simulink model "home_model"  (R2023b)
settings: Solver=VariableStepAuto  StartTime=0.0  StopTime=43200  MaxStep=0.05  RelTol=1e-3
libraries: SimscapeFluids_lib x32, fl_lib x31, nesl_utility x21
(part 1 of 2)
settings Model: Creator=jchouina  LastModifiedBy=jchouina

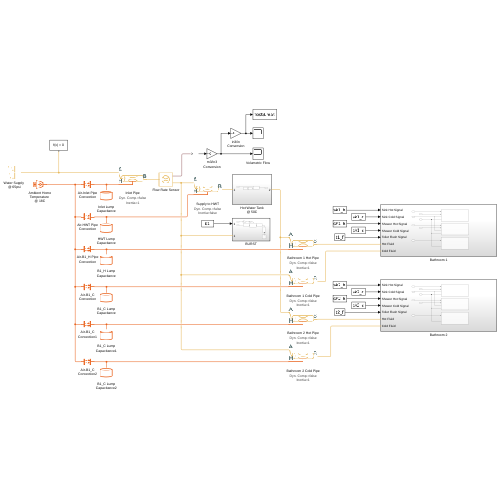
[thumbnail: Simulink's stored preview of the top-level diagram]
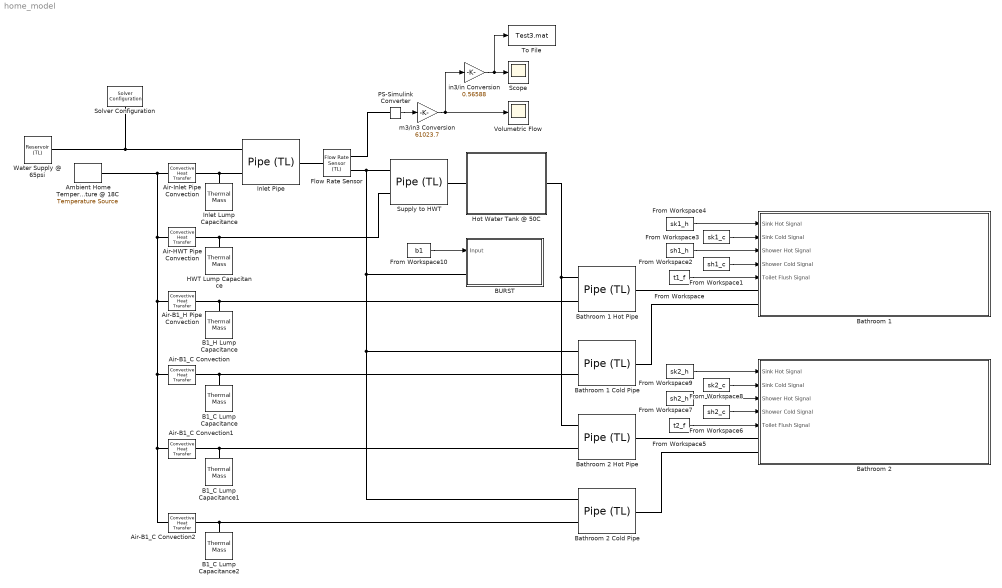
== system home_model ==
  Air-B1_C Convection : fl_lib/Thermal/Thermal Elements/Convective Heat Transfer  thermal_type=foundation.enum.constant_variable.constant  area=550 in^2  heat_tr_coeff=13.14 W/(K*m^2)  min_heat_tr_coeff=1e-3 W/(K*m^2)  T_specify=off  T_priority=None  T=0 K  T_nominal_specify=off  T_nominal_unit=K  T_nominal_value=1  Q_specify=off  Q_priority=None  Q=0 W  Q_nominal_specify=off  Q_nominal_unit=W  Q_nominal_value=1
  Air-B1_C Convection1 : fl_lib/Thermal/Thermal Elements/Convective Heat Transfer  thermal_type=foundation.enum.constant_variable.constant  area=550 in^2  heat_tr_coeff=13.14 W/(K*m^2)  min_heat_tr_coeff=1e-3 W/(K*m^2)  T_specify=off  T_priority=None  T=0 K  T_nominal_specify=off  T_nominal_unit=K  T_nominal_value=1  Q_specify=off  Q_priority=None  Q=0 W  Q_nominal_specify=off  Q_nominal_unit=W  Q_nominal_value=1
  Air-B1_C Convection2 : fl_lib/Thermal/Thermal Elements/Convective Heat Transfer  thermal_type=foundation.enum.constant_variable.constant  area=550 in^2  heat_tr_coeff=13.14 W/(K*m^2)  min_heat_tr_coeff=1e-3 W/(K*m^2)  T_specify=off  T_priority=None  T=0 K  T_nominal_specify=off  T_nominal_unit=K  T_nominal_value=1  Q_specify=off  Q_priority=None  Q=0 W  Q_nominal_specify=off  Q_nominal_unit=W  Q_nominal_value=1
  Air-B1_H Pipe Convection : fl_lib/Thermal/Thermal Elements/Convective Heat Transfer  thermal_type=foundation.enum.constant_variable.constant  area=550 in^2  heat_tr_coeff=13.14 W/(K*m^2)  min_heat_tr_coeff=1e-3 W/(K*m^2)  T_specify=off  T_priority=None  T=0 K  T_nominal_specify=off  T_nominal_unit=K  T_nominal_value=1  Q_specify=off  Q_priority=None  Q=0 W  Q_nominal_specify=off  Q_nominal_unit=W  Q_nominal_value=1
  Air-HWT Pipe Convection : fl_lib/Thermal/Thermal Elements/Convective Heat Transfer  thermal_type=foundation.enum.constant_variable.constant  area=550 in^2  heat_tr_coeff=13.14 W/(K*m^2)  min_heat_tr_coeff=1e-3 W/(K*m^2)  T_specify=off  T_priority=None  T=0 K  T_nominal_specify=off  T_nominal_unit=K  T_nominal_value=1  Q_specify=off  Q_priority=None  Q=0 W  Q_nominal_specify=off  Q_nominal_unit=W  Q_nominal_value=1
  Air-Inlet Pipe Convection : fl_lib/Thermal/Thermal Elements/Convective Heat Transfer  thermal_type=foundation.enum.constant_variable.constant  area=550 in^2  heat_tr_coeff=13.14 W/(K*m^2)  min_heat_tr_coeff=1e-3 W/(K*m^2)  T_specify=off  T_priority=None  T=0 K  T_nominal_specify=off  T_nominal_unit=K  T_nominal_value=1  Q_specify=off  Q_priority=None  Q=0 W  Q_nominal_specify=off  Q_nominal_unit=W  Q_nominal_value=1
  Ambient Home Temperature @ 18C : fl_lib/Thermal/Thermal Sources/Temperature Source  temperature=18 degC
  B1_C Lump Capacitance : fl_lib/Thermal/Thermal Elements/Thermal Mass  mass_type=foundation.enum.constant_variable.constant  mass=2.25 kg  sp_heat=390 J/(K*kg)  mass_min=1e-6 kg  num_ports=foundation.enum.numPorts2.one  m_specify=off  m_priority=High  m=1 kg  m_nominal_specify=off  m_nominal_unit=kg  m_nominal_value=1  T_specify=off  T_priority=High  T=300 K  T_nominal_specify=off  T_nominal_unit=K  T_nominal_value=1  Q_specify=off  Q_priority=None  Q=0 W  Q_nominal_specify=off  Q_nominal_unit=W  Q_nominal_value=1
  B1_C Lump Capacitance1 : fl_lib/Thermal/Thermal Elements/Thermal Mass  mass_type=foundation.enum.constant_variable.constant  mass=2.25 kg  sp_heat=390 J/(K*kg)  mass_min=1e-6 kg  num_ports=foundation.enum.numPorts2.one  m_specify=off  m_priority=High  m=1 kg  m_nominal_specify=off  m_nominal_unit=kg  m_nominal_value=1  T_specify=off  T_priority=High  T=300 K  T_nominal_specify=off  T_nominal_unit=K  T_nominal_value=1  Q_specify=off  Q_priority=None  Q=0 W  Q_nominal_specify=off  Q_nominal_unit=W  Q_nominal_value=1
  B1_C Lump Capacitance2 : fl_lib/Thermal/Thermal Elements/Thermal Mass  mass_type=foundation.enum.constant_variable.constant  mass=2.25 kg  sp_heat=390 J/(K*kg)  mass_min=1e-6 kg  num_ports=foundation.enum.numPorts2.one  m_specify=off  m_priority=High  m=1 kg  m_nominal_specify=off  m_nominal_unit=kg  m_nominal_value=1  T_specify=off  T_priority=High  T=300 K  T_nominal_specify=off  T_nominal_unit=K  T_nominal_value=1  Q_specify=off  Q_priority=None  Q=0 W  Q_nominal_specify=off  Q_nominal_unit=W  Q_nominal_value=1
  B1_H Lump Capacitance : fl_lib/Thermal/Thermal Elements/Thermal Mass  mass_type=foundation.enum.constant_variable.constant  mass=2.25 kg  sp_heat=390 J/(K*kg)  mass_min=1e-6 kg  num_ports=foundation.enum.numPorts2.one  m_specify=off  m_priority=High  m=1 kg  m_nominal_specify=off  m_nominal_unit=kg  m_nominal_value=1  T_specify=off  T_priority=High  T=300 K  T_nominal_specify=off  T_nominal_unit=K  T_nominal_value=1  Q_specify=off  Q_priority=None  Q=0 W  Q_nominal_specify=off  Q_nominal_unit=W  Q_nominal_value=1
  BURST : Subsystem
  Bathroom 1 : Subsystem
  Bathroom 1 Cold Pipe : fl_lib/Thermal Liquid/Elements/Pipe (TL)  length=360 in  area=0.442 in^2  Dh=0.75 in  length_add=0 m  roughness=1e-5 m  Re_lam=2000  Re_tur=4000  shape_factor=64  Nu_lam=3.66  dynamic_compressibility=false  inertia=1  p0=65 psi  T0=283.15 K  mdot0=0 kg/s
      settings: AttributesFormatString=|
      | Dyn. Comp.=%<dynamic_compressibility>
      | Inertia=%<inertia>
  Bathroom 1 Hot Pipe : fl_lib/Thermal Liquid/Elements/Pipe (TL)  length=360 in  area=0.442 in^2  Dh=0.75 in  length_add=0 m  roughness=1e-5 m  Re_lam=2000  Re_tur=4000  shape_factor=64  Nu_lam=3.66  dynamic_compressibility=false  inertia=1  p0=65 psi  T0=283.15 K  mdot0=0 kg/s
      settings: AttributesFormatString=|
      | Dyn. Comp.=%<dynamic_compressibility>
      | Inertia=%<inertia>
  Bathroom 2 : Subsystem
  Bathroom 2 Cold Pipe : fl_lib/Thermal Liquid/Elements/Pipe (TL)  length=440 in  area=0.442 in^2  Dh=0.75 in  length_add=0 m  roughness=1e-5 m  Re_lam=2000  Re_tur=4000  shape_factor=64  Nu_lam=3.66  dynamic_compressibility=false  inertia=1  p0=65 psi  T0=283.15 K  mdot0=0 kg/s
      settings: AttributesFormatString=|
      | Dyn. Comp.=%<dynamic_compressibility>
      | Inertia=%<inertia>
  Bathroom 2 Hot Pipe : fl_lib/Thermal Liquid/Elements/Pipe (TL)  length=440 in  area=0.442 in^2  Dh=0.75 in  length_add=0 m  roughness=1e-5 m  Re_lam=2000  Re_tur=4000  shape_factor=64  Nu_lam=3.66  dynamic_compressibility=false  inertia=1  p0=65 psi  T0=283.15 K  mdot0=0 kg/s
      settings: AttributesFormatString=|
      | Dyn. Comp.=%<dynamic_compressibility>
      | Inertia=%<inertia>
  "Flow Rate Sensor " : fl_lib/Thermal Liquid/Sensors/Flow Rate Sensor (TL)  mass_flow_measure=false  volumetric_flow_measure=true  energy_flow_measure=false
      settings: InternalSimscapePortConfiguration="{\"Bottom\":[],\"Left\":[{\"id\":\"A\",\"label\":\"A\",\"type\":\"foundation.thermal_liquid.thermal_liquid\"}],\"Right\":[{\"id\":\"B\",\"label\":\"B\",\"type\":\"foundation.thermal_liquid.thermal_liquid\"},{\"id\":\"V\",\"label\":\"V\",\"type\":\"output\"}],\"Top\":[]}"
  From Workspace : FromWorkspace  VariableName=t1_f  SampleTime=-1
  From Workspace1 : FromWorkspace  VariableName=sh1_c  SampleTime=-1
  From Workspace10 : FromWorkspace  VariableName=b1
  From Workspace2 : FromWorkspace  VariableName=sh1_h  SampleTime=-1
  From Workspace3 : FromWorkspace  VariableName=sk1_c  SampleTime=-1
  From Workspace4 : FromWorkspace  VariableName=sk1_h  SampleTime=-1
  From Workspace5 : FromWorkspace  VariableName=t2_f  SampleTime=-1
  From Workspace6 : FromWorkspace  VariableName=sh2_c  SampleTime=-1
  From Workspace7 : FromWorkspace  VariableName=sh2_h  SampleTime=-1
  From Workspace8 : FromWorkspace  VariableName=sk2_c  SampleTime=-1
  From Workspace9 : FromWorkspace  VariableName=sk2_h  SampleTime=-1
  HWT Lump Capacitance : fl_lib/Thermal/Thermal Elements/Thermal Mass  mass_type=foundation.enum.constant_variable.constant  mass=2.25 kg  sp_heat=390 J/(K*kg)  mass_min=1e-6 kg  num_ports=foundation.enum.numPorts2.one  m_specify=off  m_priority=High  m=1 kg  m_nominal_specify=off  m_nominal_unit=kg  m_nominal_value=1  T_specify=off  T_priority=High  T=300 K  T_nominal_specify=off  T_nominal_unit=K  T_nominal_value=1  Q_specify=off  Q_priority=None  Q=0 W  Q_nominal_specify=off  Q_nominal_unit=W  Q_nominal_value=1
  Hot Water Tank @ 50C : Subsystem
  Inlet Lump Capacitance : fl_lib/Thermal/Thermal Elements/Thermal Mass  mass_type=foundation.enum.constant_variable.constant  mass=4.5 kg  sp_heat=390 J/(K*kg)  mass_min=1e-6 kg  num_ports=foundation.enum.numPorts2.one  m_specify=off  m_priority=High  m=1 kg  m_nominal_specify=off  m_nominal_unit=kg  m_nominal_value=1  T_specify=off  T_priority=High  T=300 K  T_nominal_specify=off  T_nominal_unit=K  T_nominal_value=1  Q_specify=off  Q_priority=None  Q=0 W  Q_nominal_specify=off  Q_nominal_unit=W  Q_nominal_value=1
  Inlet Pipe : fl_lib/Thermal Liquid/Elements/Pipe (TL)  length=200 in  area=0.442 in^2  Dh=0.75 in  length_add=0 m  roughness=1e-5 m  Re_lam=2000  Re_tur=4000  shape_factor=64  Nu_lam=3.66  dynamic_compressibility=false  inertia=1  p0=65 psi  T0=283.15 K  mdot0=0 kg/s
      settings: AttributesFormatString=|
      | Dyn. Comp.=%<dynamic_compressibility>
      | Inertia=%<inertia>
  PS-Simulink Converter : nesl_utility/PS-Simulink Converter  PhysicalDomain=network_engine_domain  SubClassName=ps_output  LeftPortType=input  RightPortType=output  PseudoPeriodic=off  Frequencies=[]  VectorFormat=inherit  Unit=inherit  AffineConversion=off
  Scope : Scope
  Solver Configuration : nesl_utility/Solver Configuration  PhysicalDomain=network_engine_domain  SubClassName=solver  LeftPortType=input  RightPortType=generic  Tones=[]  Harmonics=[]  SimulateNoise=off  Profile=off  UseLocalSampling=off  EnableSwitchedLinearOptims=on  FrequencyDomain=off  UseCCode=off  RelTol=0.001  AbsTol=0.001  MinStep=1e-09  ToWorkspace=off  RevertToSquareIcSolve=off  NumHomotopyIterations=100  PhasorMode=off  PhasorModeNumHarmonics=1  ConsistencySolver=NEWTON_XTOL_AFTER_FTOL  IndexReductionMethod=DerivativeReplacement  DoDC=off  ResidualTolerance=1e-09  ConsistencyTolSource=GLOBAL  ConsistencyAbsTol=0.001  ConsistencyRelTol=0.001  ConsistencyTolFactor=0.001  UseLocalSolver=off  LocalSolverChoice=NE_BACKWARD_EULER_ADVANCER  ResolveIndetEquations=on  FunctionEvalNumThread=1  LocalSolverSampleTime=0.001  DoFixedCost=off  MaxNonlinIter=3  MaxModeIter=2  ComputeImpulses=off  ImpulseIterations=2  LinearAlgebra=auto  LinearAlgebraNumThread=0  EquationFormulation=NE_TIME_EF  DelaysMemoryBudget=1024  AutomaticFiltering=on  FilteringTimeConstant=0.001  PartitionStorageMethod=AS_NEEDED  PartitionMemoryBudget=1024  PartitionMethod=ROBUST  MultibodyUseLocalSolver=off  MultibodyLocalSolverChoice=ODE1  MultibodyLocalSolverSampleTime=0.001
  Supply to HWT : fl_lib/Thermal Liquid/Elements/Pipe (TL)  length=100 in  area=0.442 in^2  Dh=0.75 in  length_add=0 m  roughness=1e-5 m  Re_lam=2000  Re_tur=4000  shape_factor=64  Nu_lam=3.66  dynamic_compressibility=false  inertia=false  p0=1 atm  T0=283.15 K  mdot0=0 kg/s
      settings: AttributesFormatString=|
      | Dyn. Comp.=%<dynamic_compressibility>
      | Inertia=%<inertia>
  To File : ToFile  Filename=Test3.mat  MatrixName=linRate  SaveFormat=Timeseries
  Volumetric Flow : Scope
  Water Supply @ 65psi : fl_lib/Thermal Liquid/Elements/Reservoir (TL)  pressure_spec=foundation.enum.pressure_spec.specified  reservoir_pressure=65 psi  reservoir_temperature=283.15 K  area=0.442 in^2
  in3/in Conversion : Gain  Gain=0.56588
  m3/in3 Conversion : Gain  Gain=61023.7
  wires:
  From Workspace/1 -> Bathroom 1/5(Toilet Flush Signal)
  From Workspace1/1 -> Bathroom 1/4(Shower Cold Signal)
  From Workspace2/1 -> Bathroom 1/3(Shower Hot Signal)
  From Workspace4/1 -> Bathroom 1/1(Sink Hot Signal)
  From Workspace3/1 -> Bathroom 1/2(Sink Cold Signal)
  From Workspace9/1 -> Bathroom 2/1(Sink Hot Signal)
  From Workspace7/1 -> Bathroom 2/3(Shower Hot Signal)
  From Workspace6/1 -> Bathroom 2/4(Shower Cold Signal)
  From Workspace8/1 -> Bathroom 2/2(Sink Cold Signal)
  From Workspace5/1 -> Bathroom 2/5(Toilet Flush Signal)
  PS-Simulink Converter/1 -> m3/in3 Conversion/1
  m3/in3 Conversion/1 -> in3/in Conversion/1, Volumetric Flow/1
  in3/in Conversion/1 -> To File/1, Scope/1
  From Workspace10/1 -> BURST/1(Input)
  connections:
  Air-Inlet Pipe Convection/RConn1 -- Inlet Pipe/LConn2 -- Inlet Lump Capacitance/LConn1
  Water Supply @ 65psi/LConn1 -- Solver Configuration/RConn1 -- Inlet Pipe/LConn1
  "Flow Rate Sensor "/LConn1 -- Inlet Pipe/RConn1
  PS-Simulink Converter/LConn1 -- "Flow Rate Sensor "/RConn2
  Air-Inlet Pipe Convection/LConn1 -- Air-B1_H Pipe Convection/LConn1 -- Air-B1_C Convection/LConn1 -- Air-B1_C Convection1/LConn1 -- Air-B1_C Convection2/LConn1 -- Air-HWT Pipe Convection/LConn1 -- Ambient Home Temperature @ 18C/LConn1
  Bathroom 1 Cold Pipe/LConn1 -- Supply to HWT/LConn1 -- "Flow Rate Sensor "/RConn1 -- BURST/LConn1 -- Bathroom 2 Cold Pipe/LConn1
  Supply to HWT/LConn2 -- Air-HWT Pipe Convection/RConn1 -- HWT Lump Capacitance/LConn1
  Bathroom 1/LConn2 -- Bathroom 1 Cold Pipe/RConn1
  Air-B1_C Convection/RConn1 -- B1_C Lump Capacitance/LConn1 -- Bathroom 1 Cold Pipe/LConn2
  Bathroom 1 Hot Pipe/LConn1 -- Hot Water Tank @ 50C/RConn1 -- Bathroom 2 Hot Pipe/LConn1
  Air-B1_H Pipe Convection/RConn1 -- Bathroom 1 Hot Pipe/LConn2 -- B1_H Lump Capacitance/LConn1
  Bathroom 1 Hot Pipe/RConn1 -- Bathroom 1/LConn1
  Hot Water Tank @ 50C/LConn1 -- Supply to HWT/RConn1
  B1_C Lump Capacitance1/LConn1 -- Bathroom 2 Hot Pipe/LConn2 -- Air-B1_C Convection1/RConn1
  B1_C Lump Capacitance2/LConn1 -- Bathroom 2 Cold Pipe/LConn2 -- Air-B1_C Convection2/RConn1
  Bathroom 2/LConn2 -- Bathroom 2 Cold Pipe/RConn1
  Bathroom 2/LConn1 -- Bathroom 2 Hot Pipe/RConn1

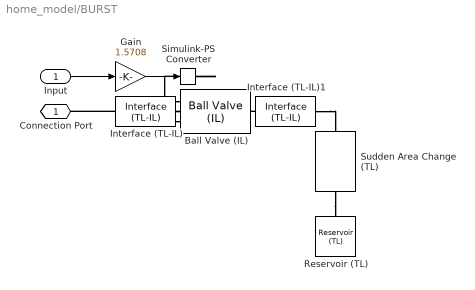
== system home_model/BURST ==
  Input : Inport
  Ball Valve (IL) : SimscapeFluids_lib/Isothermal Liquid/Valves & Orifices/Flow Control Valves/Ball Valve (IL)  valve_type=fluids.isothermal_liquid.valves_orifices.flow_control_valves.enum.BallValveSpec.Standard  parameterization=fluids.isothermal_liquid.valves_orifices.flow_control_valves.enum.FlowCoefficientSpec.Kv  Cv_max=32 gpm  Kv_max=49 m^3/hr  Cd=0.64  area_port=pi * (25 ^ 2) / 4 mm^2  area_ball=pi * (20 ^ 2) / 4 mm^2  Cv_TLU=[1e-06, .58, 1.15, 1.9, 2.8, 4.3, 7, 10.5, 17, 26, 32] gpm  Kv_TLU=[1e-06, .34, .76, 1.6, 2.45, 4.1, 5.75, 9.4, 13, 28, 50] m^3/hr  area_TLU=[1e-10, 62.5, 125, 187.5, 250, 312.5, 375, 437.5, 500, 562.5, 625] mm^2  rotation_TLU=pi / 2 .* [0, .1, .2, .3, .4, .5, .6, .7, .8, .9, 1] rad  area_leak=1e-10 m^2  Re_c=150  rho_water60F=0.99897 g/cm^3  rho_water15C=0.99913 g/cm^3
      settings: InternalSimscapePortConfiguration="{\"Bottom\":[],\"Left\":[{\"id\":\"A\",\"label\":\"A\",\"type\":\"foundation.isothermal_liquid.isothermal_liquid\"}],\"Right\":[{\"id\":\"B\",\"label\":\"B\",\"type\":\"foundation.isothermal_liquid.isothermal_liquid\"}],\"Top\":[{\"id\":\"S\",\"label\":\"S\",\"type\":\"input\"}]}"
  Gain : Gain  Gain=1.5708
  Interface (TL-IL) : SimscapeFluids_lib/Fluid Network Interfaces/Interface (TL-IL)  interface_domain_spec=fluids.interfaces.enum.interface_domain_spec.TL_IL  temperature_spec=foundation.enum.constant_controlled.constant  T_interface=293.15 K  area_TL=0.01 m^2
      settings: InternalSimscapePortConfiguration="{\"Bottom\":[],\"Left\":[{\"id\":\"TL\",\"label\":\"TL\",\"type\":\"foundation.thermal_liquid.thermal_liquid\"}],\"Right\":[{\"id\":\"IL\",\"label\":\"IL\",\"type\":\"foundation.isothermal_liquid.isothermal_liquid\"}],\"Top\":[]}"
  Interface (TL-IL)1 : SimscapeFluids_lib/Fluid Network Interfaces/Interface (TL-IL)  interface_domain_spec=fluids.interfaces.enum.interface_domain_spec.TL_IL  temperature_spec=foundation.enum.constant_controlled.constant  T_interface=293.15 K  area_TL=0.01 m^2
      settings: InternalSimscapePortConfiguration="{\"Bottom\":[],\"Left\":[{\"id\":\"TL\",\"label\":\"TL\",\"type\":\"foundation.thermal_liquid.thermal_liquid\"}],\"Right\":[{\"id\":\"IL\",\"label\":\"IL\",\"type\":\"foundation.isothermal_liquid.isothermal_liquid\"}],\"Top\":[]}"
  Reservoir (TL) : fl_lib/Thermal Liquid/Elements/Reservoir (TL)  pressure_spec=foundation.enum.pressure_spec.atmospheric  reservoir_pressure=0.101325 MPa  reservoir_temperature=293.15 K  area=0.01 m^2
  Simulink-PS Converter : nesl_utility/Simulink-PS Converter  PhysicalDomain=network_engine_domain  SubClassName=ps_input  LeftPortType=input  RightPortType=output  PseudoPeriodic=off  Frequencies=[]  NoiseDistribution=none  NoiseParameters=[]  Unit=1  AffineConversion=off  FilteringAndDerivatives=provide  SimscapeFilterOrder=1  InputFilterTimeConstant=0.001  UdotUserProvided=0
  Sudden Area Change (TL) : SimscapeFluids_lib/Thermal Liquid/Pipes & Fittings/Sudden Area Change (TL)  loss_spec=fluids.thermal_liquid.enum.area_change_loss_spec.empirical  area_A=0.442 m^2  area_B=10 in^2  K_c=1  K_e=1  Re_TLU=[10, 20, 30, 40, 50, 100, 200, 500, 1000, 2000]  loss_contraction_TLU=[5, 2.7, 1.8, 1.46, 1.3, .9, .65, .42, .3, .2]  loss_expansion_TLU=[3.1, 2.3, 1.65, 1.35, 1.15, .9, .75, .65, .9, .65]  Re_critical=150
      settings: InternalSimscapePortConfiguration="{\"Bottom\":[],\"Left\":[{\"id\":\"A\",\"label\":\"A\",\"type\":\"foundation.thermal_liquid.thermal_liquid\"}],\"Right\":[{\"id\":\"B\",\"label\":\"B\",\"type\":\"foundation.thermal_liquid.thermal_liquid\"}],\"Top\":[]}"
  Connection Port : PMIOPort  Side=Left
  wires:
  Input/1 -> Gain/1
  Gain/1 -> Simulink-PS Converter/1
  connections:
  Interface (TL-IL)/RConn1 -- Ball Valve (IL)/LConn1
  Simulink-PS Converter/RConn1 -- Ball Valve (IL)/LConn2
  Interface (TL-IL)/LConn1 -- Connection Port/RConn1
  Sudden Area Change (TL)/RConn1 -- Reservoir (TL)/LConn1
  Interface (TL-IL)1/LConn1 -- Sudden Area Change (TL)/LConn1
  Interface (TL-IL)1/RConn1 -- Ball Valve (IL)/RConn1

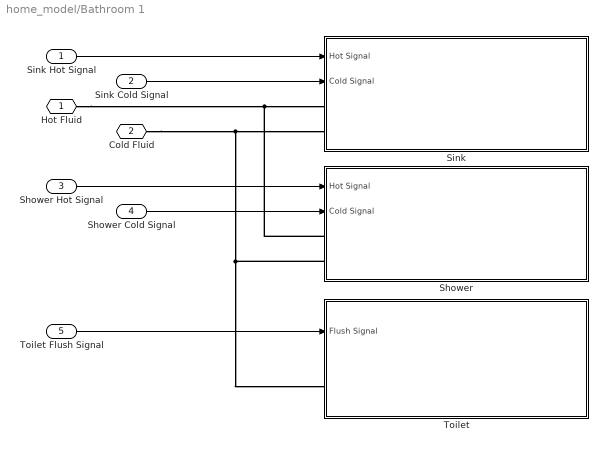
== system home_model/Bathroom 1 ==
  Sink Hot Signal : Inport
  Sink Cold Signal : Inport  Port=2
  Shower Hot Signal : Inport  Port=3
  Shower Cold Signal : Inport  Port=4
  Toilet Flush Signal : Inport  Port=5
  Shower : Subsystem
  Sink : Subsystem
  Toilet : Subsystem
  Hot Fluid : PMIOPort  Side=Left
  Cold Fluid : PMIOPort  Port=2  Side=Left
  wires:
  Sink Hot Signal/1 -> Sink/1(Hot Signal)
  Sink Cold Signal/1 -> Sink/2(Cold Signal)
  Shower Cold Signal/1 -> Shower/2(Cold Signal)
  Shower Hot Signal/1 -> Shower/1(Hot Signal)
  Toilet Flush Signal/1 -> Toilet/1(Flush Signal)
  connections:
  Hot Fluid/RConn1 -- Shower/LConn1 -- Sink/LConn1
  Cold Fluid/RConn1 -- Sink/LConn2 -- Toilet/LConn1 -- Shower/LConn2

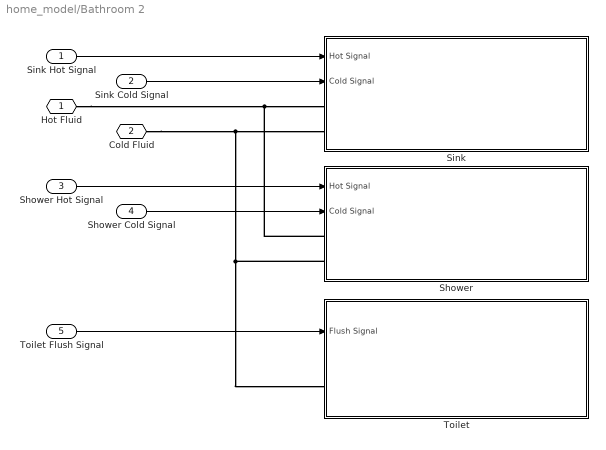
== system home_model/Bathroom 2 ==
  Sink Hot Signal : Inport
  Sink Cold Signal : Inport  Port=2
  Shower Hot Signal : Inport  Port=3
  Shower Cold Signal : Inport  Port=4
  Toilet Flush Signal : Inport  Port=5
  Shower : Subsystem
  Sink : Subsystem
  Toilet : Subsystem
  Hot Fluid : PMIOPort  Side=Left
  Cold Fluid : PMIOPort  Port=2  Side=Left
  wires:
  Sink Hot Signal/1 -> Sink/1(Hot Signal)
  Sink Cold Signal/1 -> Sink/2(Cold Signal)
  Shower Cold Signal/1 -> Shower/2(Cold Signal)
  Shower Hot Signal/1 -> Shower/1(Hot Signal)
  Toilet Flush Signal/1 -> Toilet/1(Flush Signal)
  connections:
  Hot Fluid/RConn1 -- Shower/LConn1 -- Sink/LConn1
  Cold Fluid/RConn1 -- Sink/LConn2 -- Toilet/LConn1 -- Shower/LConn2

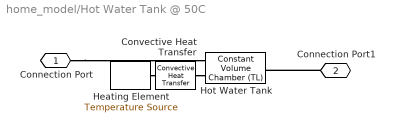
== system home_model/Hot Water Tank @ 50C ==
  Convective Heat Transfer : fl_lib/Thermal/Thermal Elements/Convective Heat Transfer  thermal_type=foundation.enum.constant_variable.constant  area=0.135 m^2  heat_tr_coeff=800 W/(K*m^2)  min_heat_tr_coeff=1e-3 W/(K*m^2)  T_specify=off  T_priority=None  T=0 K  T_nominal_specify=off  T_nominal_unit=K  T_nominal_value=1  Q_specify=off  Q_priority=None  Q=0 W  Q_nominal_specify=off  Q_nominal_unit=W  Q_nominal_value=1
  Heating Element : fl_lib/Thermal/Thermal Sources/Temperature Source  temperature=50 degC
  Hot Water Tank : fl_lib/Thermal Liquid/Elements/Constant Volume Chamber (TL)  volume=40 gal  num_ports=foundation.enum.num_ports.two  area_A=0.442 in^2  area_B=0.442 in^2  area_C=0.01 m^2  area_D=0.01 m^2  p_I_specify=off  p_I_priority=High  p_I=0.101325 MPa  p_I_nominal_specify=off  p_I_nominal_unit=MPa  p_I_nominal_value=1  T_I_specify=off  T_I_priority=High  T_I=293.15 K  T_I_nominal_specify=off  T_I_nominal_unit=K  T_I_nominal_value=1  u_I_specify=off  u_I_priority=None  u_I=83.906 kJ/kg  u_I_nominal_specify=off  u_I_nominal_unit=kJ/kg  u_I_nominal_value=1  rho_I_specify=off  rho_I_priority=None  rho_I=998.21 kg/m^3  rho_I_nominal_specify=off  rho_I_nominal_unit=kg/m^3  rho_I_nominal_value=1
      settings: InternalSimscapePortConfiguration="{\"Bottom\":[],\"Left\":[{\"id\":\"A\",\"label\":\"A\",\"type\":\"foundation.thermal_liquid.thermal_liquid\"},{\"id\":\"H\",\"label\":\"H\",\"type\":\"foundation.thermal.thermal\"}],\"Right\":[{\"id\":\"B\",\"label\":\"B\",\"type\":\"foundation.thermal_liquid.thermal_liquid\"}],\"Top\":[]}"
  Connection Port : PMIOPort  Side=Left
  Connection Port1 : PMIOPort  Port=2  Side=Right
  connections:
  Heating Element/LConn1 -- Convective Heat Transfer/LConn1
  Convective Heat Transfer/RConn1 -- Hot Water Tank/LConn2
  Connection Port/RConn1 -- Hot Water Tank/LConn1
  Connection Port1/RConn1 -- Hot Water Tank/RConn1

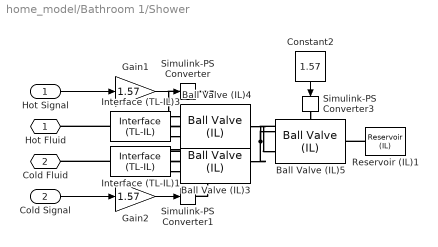
== system home_model/Bathroom 1/Shower ==
  Hot Signal : Inport
  Cold Signal : Inport  Port=2
  Ball Valve (IL)3 : SimscapeFluids_lib/Isothermal Liquid/Valves & Orifices/Flow Control Valves/Ball Valve (IL)  valve_type=fluids.isothermal_liquid.valves_orifices.flow_control_valves.enum.BallValveSpec.Standard  parameterization=fluids.isothermal_liquid.valves_orifices.flow_control_valves.enum.FlowCoefficientSpec.Kv  Cv_max=32 gpm  Kv_max=2 gpm  Cd=0.64  area_port=pi * (75 ^ 2) / 4 mm^2  area_ball=pi * (75 ^ 2) / 4 mm^2  Cv_TLU=[1e-06, .58, 1.15, 1.9, 2.8, 4.3, 7, 10.5, 17, 26, 32] gpm  Kv_TLU=[1e-06, .34, .76, 1.6, 2.45, 4.1, 5.75, 9.4, 13, 28, 50] m^3/hr  area_TLU=[1e-10, 62.5, 125, 187.5, 250, 312.5, 375, 437.5, 500, 562.5, 625] mm^2  rotation_TLU=pi / 2 .* [0, .1, .2, .3, .4, .5, .6, .7, .8, .9, 1] rad  area_leak=1e-10 m^2  Re_c=150  rho_water60F=0.99897 g/cm^3  rho_water15C=0.99913 g/cm^3
      settings: InternalSimscapePortConfiguration="{\"Bottom\":[],\"Left\":[{\"id\":\"A\",\"label\":\"A\",\"type\":\"foundation.isothermal_liquid.isothermal_liquid\"}],\"Right\":[{\"id\":\"B\",\"label\":\"B\",\"type\":\"foundation.isothermal_liquid.isothermal_liquid\"}],\"Top\":[{\"id\":\"S\",\"label\":\"S\",\"type\":\"input\"}]}"
  Ball Valve (IL)4 : SimscapeFluids_lib/Isothermal Liquid/Valves & Orifices/Flow Control Valves/Ball Valve (IL)  valve_type=fluids.isothermal_liquid.valves_orifices.flow_control_valves.enum.BallValveSpec.Standard  parameterization=fluids.isothermal_liquid.valves_orifices.flow_control_valves.enum.FlowCoefficientSpec.Kv  Cv_max=32 gpm  Kv_max=2 gpm  Cd=0.64  area_port=pi * (75 ^ 2) / 4 mm^2  area_ball=pi * (75 ^ 2) / 4 mm^2  Cv_TLU=[1e-06, .58, 1.15, 1.9, 2.8, 4.3, 7, 10.5, 17, 26, 32] gpm  Kv_TLU=[1e-06, .34, .76, 1.6, 2.45, 4.1, 5.75, 9.4, 13, 28, 50] m^3/hr  area_TLU=[1e-10, 62.5, 125, 187.5, 250, 312.5, 375, 437.5, 500, 562.5, 625] mm^2  rotation_TLU=pi / 2 .* [0, .1, .2, .3, .4, .5, .6, .7, .8, .9, 1] rad  area_leak=1e-10 m^2  Re_c=150  rho_water60F=0.99897 g/cm^3  rho_water15C=0.99913 g/cm^3
      settings: InternalSimscapePortConfiguration="{\"Bottom\":[],\"Left\":[{\"id\":\"A\",\"label\":\"A\",\"type\":\"foundation.isothermal_liquid.isothermal_liquid\"}],\"Right\":[{\"id\":\"B\",\"label\":\"B\",\"type\":\"foundation.isothermal_liquid.isothermal_liquid\"}],\"Top\":[{\"id\":\"S\",\"label\":\"S\",\"type\":\"input\"}]}"
  Ball Valve (IL)5 : SimscapeFluids_lib/Isothermal Liquid/Valves & Orifices/Flow Control Valves/Ball Valve (IL)  valve_type=fluids.isothermal_liquid.valves_orifices.flow_control_valves.enum.BallValveSpec.Standard  parameterization=fluids.isothermal_liquid.valves_orifices.flow_control_valves.enum.FlowCoefficientSpec.Kv  Cv_max=32 gpm  Kv_max=2 gpm  Cd=0.64  area_port=pi * (25 ^ 2) / 4 mm^2  area_ball=pi * (20 ^ 2) / 4 mm^2  Cv_TLU=[1e-06, .58, 1.15, 1.9, 2.8, 4.3, 7, 10.5, 17, 26, 32] gpm  Kv_TLU=[1e-06, .34, .76, 1.6, 2.45, 4.1, 5.75, 9.4, 13, 28, 50] m^3/hr  area_TLU=[1e-10, 62.5, 125, 187.5, 250, 312.5, 375, 437.5, 500, 562.5, 625] mm^2  rotation_TLU=pi / 2 .* [0, .1, .2, .3, .4, .5, .6, .7, .8, .9, 1] rad  area_leak=1e-10 m^2  Re_c=150  rho_water60F=0.99897 g/cm^3  rho_water15C=0.99913 g/cm^3
      settings: InternalSimscapePortConfiguration="{\"Bottom\":[],\"Left\":[{\"id\":\"A\",\"label\":\"A\",\"type\":\"foundation.isothermal_liquid.isothermal_liquid\"}],\"Right\":[{\"id\":\"B\",\"label\":\"B\",\"type\":\"foundation.isothermal_liquid.isothermal_liquid\"}],\"Top\":[{\"id\":\"S\",\"label\":\"S\",\"type\":\"input\"}]}"
  Constant2 : Constant  Value=1.57
  Gain1 : Gain  Gain=1.57
  Gain2 : Gain  Gain=1.57
  Interface (TL-IL)1 : SimscapeFluids_lib/Fluid Network Interfaces/Interface (TL-IL)  interface_domain_spec=fluids.interfaces.enum.interface_domain_spec.TL_IL  temperature_spec=foundation.enum.constant_controlled.constant  T_interface=293.15 K  area_TL=0.01 m^2
      settings: InternalSimscapePortConfiguration="{\"Bottom\":[],\"Left\":[{\"id\":\"TL\",\"label\":\"TL\",\"type\":\"foundation.thermal_liquid.thermal_liquid\"}],\"Right\":[{\"id\":\"IL\",\"label\":\"IL\",\"type\":\"foundation.isothermal_liquid.isothermal_liquid\"}],\"Top\":[]}"
  Interface (TL-IL)3 : SimscapeFluids_lib/Fluid Network Interfaces/Interface (TL-IL)  interface_domain_spec=fluids.interfaces.enum.interface_domain_spec.TL_IL  temperature_spec=foundation.enum.constant_controlled.constant  T_interface=293.15 K  area_TL=0.01 m^2
      settings: InternalSimscapePortConfiguration="{\"Bottom\":[],\"Left\":[{\"id\":\"TL\",\"label\":\"TL\",\"type\":\"foundation.thermal_liquid.thermal_liquid\"}],\"Right\":[{\"id\":\"IL\",\"label\":\"IL\",\"type\":\"foundation.isothermal_liquid.isothermal_liquid\"}],\"Top\":[]}"
  Reservoir (IL)1 : fl_lib/Isothermal Liquid/Elements/Reservoir (IL)  reservoir_type=foundation.enum.constant_controlled.constant  pressure_spec=foundation.enum.pressure_spec.atmospheric  reservoir_pressure=0.101325 MPa
  Simulink-PS Converter : nesl_utility/Simulink-PS Converter  PhysicalDomain=network_engine_domain  SubClassName=ps_input  LeftPortType=input  RightPortType=output  PseudoPeriodic=off  Frequencies=[]  NoiseDistribution=none  NoiseParameters=[]  Unit=1  AffineConversion=off  FilteringAndDerivatives=provide  SimscapeFilterOrder=1  InputFilterTimeConstant=0.001  UdotUserProvided=0
  Simulink-PS Converter1 : nesl_utility/Simulink-PS Converter  PhysicalDomain=network_engine_domain  SubClassName=ps_input  LeftPortType=input  RightPortType=output  PseudoPeriodic=off  Frequencies=[]  NoiseDistribution=none  NoiseParameters=[]  Unit=1  AffineConversion=off  FilteringAndDerivatives=provide  SimscapeFilterOrder=1  InputFilterTimeConstant=0.001  UdotUserProvided=0
  Simulink-PS Converter3 : nesl_utility/Simulink-PS Converter  PhysicalDomain=network_engine_domain  SubClassName=ps_input  LeftPortType=input  RightPortType=output  PseudoPeriodic=off  Frequencies=[]  NoiseDistribution=none  NoiseParameters=[]  Unit=1  AffineConversion=off  FilteringAndDerivatives=provide  SimscapeFilterOrder=1  InputFilterTimeConstant=0.001  UdotUserProvided=0
  Hot Fluid : PMIOPort  Side=Left
  Cold Fluid : PMIOPort  Port=2  Side=Left
  wires:
  Cold Signal/1 -> Gain2/1
  Gain2/1 -> Simulink-PS Converter1/1
  Gain1/1 -> Simulink-PS Converter/1
  Hot Signal/1 -> Gain1/1
  Constant2/1 -> Simulink-PS Converter3/1
  connections:
  Ball Valve (IL)3/LConn2 -- Simulink-PS Converter1/RConn1
  Simulink-PS Converter/RConn1 -- Ball Valve (IL)4/LConn2
  Interface (TL-IL)1/RConn1 -- Ball Valve (IL)3/LConn1
  Interface (TL-IL)1/LConn1 -- Cold Fluid/RConn1
  Interface (TL-IL)3/RConn1 -- Ball Valve (IL)4/LConn1
  Interface (TL-IL)3/LConn1 -- Hot Fluid/RConn1
  Reservoir (IL)1/LConn1 -- Ball Valve (IL)5/RConn1
  Simulink-PS Converter3/RConn1 -- Ball Valve (IL)5/LConn2
  Ball Valve (IL)4/RConn1 -- Ball Valve (IL)5/LConn1 -- Ball Valve (IL)3/RConn1

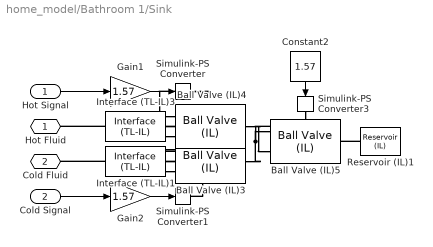
== system home_model/Bathroom 1/Sink ==
  Hot Signal : Inport
  Cold Signal : Inport  Port=2
  Ball Valve (IL)3 : SimscapeFluids_lib/Isothermal Liquid/Valves & Orifices/Flow Control Valves/Ball Valve (IL)  valve_type=fluids.isothermal_liquid.valves_orifices.flow_control_valves.enum.BallValveSpec.Standard  parameterization=fluids.isothermal_liquid.valves_orifices.flow_control_valves.enum.FlowCoefficientSpec.Kv  Cv_max=32 gpm  Kv_max=2 gpm  Cd=0.64  area_port=pi * (75 ^ 2) / 4 mm^2  area_ball=pi * (75 ^ 2) / 4 mm^2  Cv_TLU=[1e-06, .58, 1.15, 1.9, 2.8, 4.3, 7, 10.5, 17, 26, 32] gpm  Kv_TLU=[1e-06, .34, .76, 1.6, 2.45, 4.1, 5.75, 9.4, 13, 28, 50] m^3/hr  area_TLU=[1e-10, 62.5, 125, 187.5, 250, 312.5, 375, 437.5, 500, 562.5, 625] mm^2  rotation_TLU=pi / 2 .* [0, .1, .2, .3, .4, .5, .6, .7, .8, .9, 1] rad  area_leak=1e-10 m^2  Re_c=150  rho_water60F=0.99897 g/cm^3  rho_water15C=0.99913 g/cm^3
      settings: InternalSimscapePortConfiguration="{\"Bottom\":[],\"Left\":[{\"id\":\"A\",\"label\":\"A\",\"type\":\"foundation.isothermal_liquid.isothermal_liquid\"}],\"Right\":[{\"id\":\"B\",\"label\":\"B\",\"type\":\"foundation.isothermal_liquid.isothermal_liquid\"}],\"Top\":[{\"id\":\"S\",\"label\":\"S\",\"type\":\"input\"}]}"
  Ball Valve (IL)4 : SimscapeFluids_lib/Isothermal Liquid/Valves & Orifices/Flow Control Valves/Ball Valve (IL)  valve_type=fluids.isothermal_liquid.valves_orifices.flow_control_valves.enum.BallValveSpec.Standard  parameterization=fluids.isothermal_liquid.valves_orifices.flow_control_valves.enum.FlowCoefficientSpec.Kv  Cv_max=32 gpm  Kv_max=2 gpm  Cd=0.64  area_port=pi * (75 ^ 2) / 4 mm^2  area_ball=pi * (75 ^ 2) / 4 mm^2  Cv_TLU=[1e-06, .58, 1.15, 1.9, 2.8, 4.3, 7, 10.5, 17, 26, 32] gpm  Kv_TLU=[1e-06, .34, .76, 1.6, 2.45, 4.1, 5.75, 9.4, 13, 28, 50] m^3/hr  area_TLU=[1e-10, 62.5, 125, 187.5, 250, 312.5, 375, 437.5, 500, 562.5, 625] mm^2  rotation_TLU=pi / 2 .* [0, .1, .2, .3, .4, .5, .6, .7, .8, .9, 1] rad  area_leak=1e-10 m^2  Re_c=150  rho_water60F=0.99897 g/cm^3  rho_water15C=0.99913 g/cm^3
      settings: InternalSimscapePortConfiguration="{\"Bottom\":[],\"Left\":[{\"id\":\"A\",\"label\":\"A\",\"type\":\"foundation.isothermal_liquid.isothermal_liquid\"}],\"Right\":[{\"id\":\"B\",\"label\":\"B\",\"type\":\"foundation.isothermal_liquid.isothermal_liquid\"}],\"Top\":[{\"id\":\"S\",\"label\":\"S\",\"type\":\"input\"}]}"
  Ball Valve (IL)5 : SimscapeFluids_lib/Isothermal Liquid/Valves & Orifices/Flow Control Valves/Ball Valve (IL)  valve_type=fluids.isothermal_liquid.valves_orifices.flow_control_valves.enum.BallValveSpec.Standard  parameterization=fluids.isothermal_liquid.valves_orifices.flow_control_valves.enum.FlowCoefficientSpec.Kv  Cv_max=32 gpm  Kv_max=2 gpm  Cd=0.64  area_port=pi * (25 ^ 2) / 4 mm^2  area_ball=pi * (20 ^ 2) / 4 mm^2  Cv_TLU=[1e-06, .58, 1.15, 1.9, 2.8, 4.3, 7, 10.5, 17, 26, 32] gpm  Kv_TLU=[1e-06, .34, .76, 1.6, 2.45, 4.1, 5.75, 9.4, 13, 28, 50] m^3/hr  area_TLU=[1e-10, 62.5, 125, 187.5, 250, 312.5, 375, 437.5, 500, 562.5, 625] mm^2  rotation_TLU=pi / 2 .* [0, .1, .2, .3, .4, .5, .6, .7, .8, .9, 1] rad  area_leak=1e-10 m^2  Re_c=150  rho_water60F=0.99897 g/cm^3  rho_water15C=0.99913 g/cm^3
      settings: InternalSimscapePortConfiguration="{\"Bottom\":[],\"Left\":[{\"id\":\"A\",\"label\":\"A\",\"type\":\"foundation.isothermal_liquid.isothermal_liquid\"}],\"Right\":[{\"id\":\"B\",\"label\":\"B\",\"type\":\"foundation.isothermal_liquid.isothermal_liquid\"}],\"Top\":[{\"id\":\"S\",\"label\":\"S\",\"type\":\"input\"}]}"
  Constant2 : Constant  Value=1.57
  Gain1 : Gain  Gain=1.57
  Gain2 : Gain  Gain=1.57
  Interface (TL-IL)1 : SimscapeFluids_lib/Fluid Network Interfaces/Interface (TL-IL)  interface_domain_spec=fluids.interfaces.enum.interface_domain_spec.TL_IL  temperature_spec=foundation.enum.constant_controlled.constant  T_interface=293.15 K  area_TL=0.01 m^2
      settings: InternalSimscapePortConfiguration="{\"Bottom\":[],\"Left\":[{\"id\":\"TL\",\"label\":\"TL\",\"type\":\"foundation.thermal_liquid.thermal_liquid\"}],\"Right\":[{\"id\":\"IL\",\"label\":\"IL\",\"type\":\"foundation.isothermal_liquid.isothermal_liquid\"}],\"Top\":[]}"
  Interface (TL-IL)3 : SimscapeFluids_lib/Fluid Network Interfaces/Interface (TL-IL)  interface_domain_spec=fluids.interfaces.enum.interface_domain_spec.TL_IL  temperature_spec=foundation.enum.constant_controlled.constant  T_interface=293.15 K  area_TL=0.01 m^2
      settings: InternalSimscapePortConfiguration="{\"Bottom\":[],\"Left\":[{\"id\":\"TL\",\"label\":\"TL\",\"type\":\"foundation.thermal_liquid.thermal_liquid\"}],\"Right\":[{\"id\":\"IL\",\"label\":\"IL\",\"type\":\"foundation.isothermal_liquid.isothermal_liquid\"}],\"Top\":[]}"
  Reservoir (IL)1 : fl_lib/Isothermal Liquid/Elements/Reservoir (IL)  reservoir_type=foundation.enum.constant_controlled.constant  pressure_spec=foundation.enum.pressure_spec.atmospheric  reservoir_pressure=0.101325 MPa
  Simulink-PS Converter : nesl_utility/Simulink-PS Converter  PhysicalDomain=network_engine_domain  SubClassName=ps_input  LeftPortType=input  RightPortType=output  PseudoPeriodic=off  Frequencies=[]  NoiseDistribution=none  NoiseParameters=[]  Unit=1  AffineConversion=off  FilteringAndDerivatives=provide  SimscapeFilterOrder=1  InputFilterTimeConstant=0.001  UdotUserProvided=0
  Simulink-PS Converter1 : nesl_utility/Simulink-PS Converter  PhysicalDomain=network_engine_domain  SubClassName=ps_input  LeftPortType=input  RightPortType=output  PseudoPeriodic=off  Frequencies=[]  NoiseDistribution=none  NoiseParameters=[]  Unit=1  AffineConversion=off  FilteringAndDerivatives=provide  SimscapeFilterOrder=1  InputFilterTimeConstant=0.001  UdotUserProvided=0
  Simulink-PS Converter3 : nesl_utility/Simulink-PS Converter  PhysicalDomain=network_engine_domain  SubClassName=ps_input  LeftPortType=input  RightPortType=output  PseudoPeriodic=off  Frequencies=[]  NoiseDistribution=none  NoiseParameters=[]  Unit=1  AffineConversion=off  FilteringAndDerivatives=provide  SimscapeFilterOrder=1  InputFilterTimeConstant=0.001  UdotUserProvided=0
  Hot Fluid : PMIOPort  Side=Left
  Cold Fluid : PMIOPort  Port=2  Side=Left
  wires:
  Constant2/1 -> Simulink-PS Converter3/1
  Hot Signal/1 -> Gain1/1
  Gain1/1 -> Simulink-PS Converter/1
  Gain2/1 -> Simulink-PS Converter1/1
  Cold Signal/1 -> Gain2/1
  connections:
  Ball Valve (IL)3/RConn1 -- Ball Valve (IL)5/LConn1 -- Ball Valve (IL)4/RConn1
  Simulink-PS Converter3/RConn1 -- Ball Valve (IL)5/LConn2
  Reservoir (IL)1/LConn1 -- Ball Valve (IL)5/RConn1
  Interface (TL-IL)3/LConn1 -- Hot Fluid/RConn1
  Interface (TL-IL)3/RConn1 -- Ball Valve (IL)4/LConn1
  Interface (TL-IL)1/LConn1 -- Cold Fluid/RConn1
  Interface (TL-IL)1/RConn1 -- Ball Valve (IL)3/LConn1
  Simulink-PS Converter/RConn1 -- Ball Valve (IL)4/LConn2
  Ball Valve (IL)3/LConn2 -- Simulink-PS Converter1/RConn1

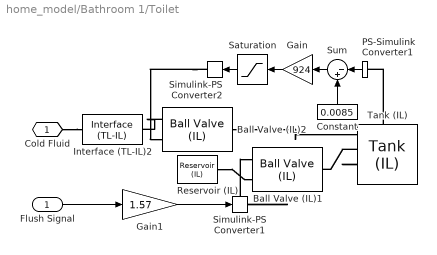
== system home_model/Bathroom 1/Toilet ==
  Flush Signal : Inport
  Ball Valve (IL)1 : SimscapeFluids_lib/Isothermal Liquid/Valves & Orifices/Flow Control Valves/Ball Valve (IL)  valve_type=fluids.isothermal_liquid.valves_orifices.flow_control_valves.enum.BallValveSpec.Standard  parameterization=fluids.isothermal_liquid.valves_orifices.flow_control_valves.enum.FlowCoefficientSpec.Kv  Cv_max=32 gpm  Kv_max=49 m^3/hr  Cd=0.64  area_port=pi * (75 ^ 2) / 4 mm^2  area_ball=pi * (75 ^ 2) / 4 mm^2  Cv_TLU=[1e-06, .58, 1.15, 1.9, 2.8, 4.3, 7, 10.5, 17, 26, 32] gpm  Kv_TLU=[1e-06, .34, .76, 1.6, 2.45, 4.1, 5.75, 9.4, 13, 28, 50] m^3/hr  area_TLU=[1e-10, 62.5, 125, 187.5, 250, 312.5, 375, 437.5, 500, 562.5, 625] mm^2  rotation_TLU=pi / 2 .* [0, .1, .2, .3, .4, .5, .6, .7, .8, .9, 1] rad  area_leak=1e-10 m^2  Re_c=150  rho_water60F=0.99897 g/cm^3  rho_water15C=0.99913 g/cm^3
      settings: InternalSimscapePortConfiguration="{\"Bottom\":[],\"Left\":[{\"id\":\"A\",\"label\":\"A\",\"type\":\"foundation.isothermal_liquid.isothermal_liquid\"}],\"Right\":[{\"id\":\"B\",\"label\":\"B\",\"type\":\"foundation.isothermal_liquid.isothermal_liquid\"}],\"Top\":[{\"id\":\"S\",\"label\":\"S\",\"type\":\"input\"}]}"
  Ball Valve (IL)2 : SimscapeFluids_lib/Isothermal Liquid/Valves & Orifices/Flow Control Valves/Ball Valve (IL)  valve_type=fluids.isothermal_liquid.valves_orifices.flow_control_valves.enum.BallValveSpec.Standard  parameterization=fluids.isothermal_liquid.valves_orifices.flow_control_valves.enum.FlowCoefficientSpec.Kv  Cv_max=32 gpm  Kv_max=2.25 gpm  Cd=0.64  area_port=pi * (9.525 ^ 2) / 4 mm^2  area_ball=pi * (9.525 ^ 2) / 4 mm^2  Cv_TLU=[1e-06, .58, 1.15, 1.9, 2.8, 4.3, 7, 10.5, 17, 26, 32] gpm  Kv_TLU=[1e-06, .34, .76, 1.6, 2.45, 4.1, 5.75, 9.4, 13, 28, 50] m^3/hr  area_TLU=[1e-10, 62.5, 125, 187.5, 250, 312.5, 375, 437.5, 500, 562.5, 625] mm^2  rotation_TLU=pi / 2 .* [0, .1, .2, .3, .4, .5, .6, .7, .8, .9, 1] rad  area_leak=1e-10 m^2  Re_c=150  rho_water60F=0.99897 g/cm^3  rho_water15C=0.99913 g/cm^3
      settings: InternalSimscapePortConfiguration="{\"Bottom\":[],\"Left\":[{\"id\":\"A\",\"label\":\"A\",\"type\":\"foundation.isothermal_liquid.isothermal_liquid\"}],\"Right\":[{\"id\":\"B\",\"label\":\"B\",\"type\":\"foundation.isothermal_liquid.isothermal_liquid\"}],\"Top\":[{\"id\":\"S\",\"label\":\"S\",\"type\":\"input\"}]}"
  Constant : Constant  Value=0.0085
  Gain : Gain  Gain=924
  Gain1 : Gain  Gain=1.57
  Interface (TL-IL)2 : SimscapeFluids_lib/Fluid Network Interfaces/Interface (TL-IL)  interface_domain_spec=fluids.interfaces.enum.interface_domain_spec.TL_IL  temperature_spec=foundation.enum.constant_controlled.constant  T_interface=293.15 K  area_TL=0.01 m^2
      settings: InternalSimscapePortConfiguration="{\"Bottom\":[],\"Left\":[{\"id\":\"TL\",\"label\":\"TL\",\"type\":\"foundation.thermal_liquid.thermal_liquid\"}],\"Right\":[{\"id\":\"IL\",\"label\":\"IL\",\"type\":\"foundation.isothermal_liquid.isothermal_liquid\"}],\"Top\":[]}"
  PS-Simulink Converter1 : nesl_utility/PS-Simulink Converter  PhysicalDomain=network_engine_domain  SubClassName=ps_output  LeftPortType=input  RightPortType=output  PseudoPeriodic=off  Frequencies=[]  VectorFormat=inherit  Unit=inherit  AffineConversion=off
  Reservoir (IL) : fl_lib/Isothermal Liquid/Elements/Reservoir (IL)  reservoir_type=foundation.enum.constant_controlled.constant  pressure_spec=foundation.enum.pressure_spec.atmospheric  reservoir_pressure=0.101325 MPa
  Saturation : Saturate  UpperLimit=1.5707  LowerLimit=0
  Simulink-PS Converter1 : nesl_utility/Simulink-PS Converter  PhysicalDomain=network_engine_domain  SubClassName=ps_input  LeftPortType=input  RightPortType=output  PseudoPeriodic=off  Frequencies=[]  NoiseDistribution=none  NoiseParameters=[]  Unit=1  AffineConversion=off  FilteringAndDerivatives=provide  SimscapeFilterOrder=1  InputFilterTimeConstant=0.001  UdotUserProvided=0
  Simulink-PS Converter2 : nesl_utility/Simulink-PS Converter  PhysicalDomain=network_engine_domain  SubClassName=ps_input  LeftPortType=input  RightPortType=output  PseudoPeriodic=off  Frequencies=[]  NoiseDistribution=none  NoiseParameters=[]  Unit=1  AffineConversion=off  FilteringAndDerivatives=provide  SimscapeFilterOrder=1  InputFilterTimeConstant=0.001  UdotUserProvided=0
  Sum : Sum  Inputs=|-+
  Tank (IL) : SimscapeFluids_lib/Isothermal Liquid/Tanks & Accumulators/Tank (IL)  num_inlet=fluids.isothermal_liquid.tanks_accumulators.enum.NumInlet.Two  pressure_spec=fluids.isothermal_liquid.tanks_accumulators.enum.TankPressureSpec.Atmospheric  tank_pressure=0.101325 MPa  volume_spec=fluids.isothermal_liquid.tanks_accumulators.enum.TankVolumeSpec.Constant  tank_area=0.135 m^2  level_TLU=[0, 3, 5] m  volume_TLU=[0, 4, 6] m^3  inlet_height_A=0.1 m  inlet_area_A=0.01 m^2  inlet_height_AB=[0,0] m  inlet_area_AB=[.442,7] in^2  inlet_height_ABC=[.1, .1, .1] m  inlet_area_ABC=[.01, .01, .01] m^2  inlet_height_ABCD=0.1 * ones(1, 4) m  inlet_area_ABCD=0.01 * ones(1, 4) m^2  inlet_height_ABCDE=0.1 * ones(1, 5) m  inlet_area_ABCDE=0.01 * ones(1, 5) m^2  inlet_height_ABCDEF=0.1 * ones(1, 6) m  inlet_area_ABCDEF=0.01 * ones(1, 6) m^2  level_check=simscape.enum.assert.action.none  capacity_check=simscape.enum.assert.action.none  max_capacity=10 m^3  g=9.81 m/s^2  level_specify=off  level_priority=High  level=5 m  level_nominal_specify=off  level_nominal_unit=m  level_nominal_value=1  volume_specify=on  volume_priority=High  volume=2 gal  volume_nominal_specify=off  volume_nominal_unit=m^3  volume_nominal_value=1  mass_specify=off  mass_priority=None  mass=5000 kg  mass_nominal_specify=off  mass_nominal_unit=kg  mass_nominal_value=1
      settings: InternalSimscapePortConfiguration="{\"Bottom\":[],\"Left\":[{\"id\":\"A\",\"label\":\"A\",\"type\":\"foundation.isothermal_liquid.isothermal_liquid\"},{\"id\":\"B\",\"label\":\"B\",\"type\":\"foundation.isothermal_liquid.isothermal_liquid\"}],\"Right\":[],\"Top\":[{\"id\":\"V\",\"label\":\"V\",\"type\":\"output\"},{\"id\":\"L\",\"label\":\"L\",\"type\":\"output\"}]}"
  Cold Fluid : PMIOPort  Side=Left
  wires:
  Flush Signal/1 -> Gain1/1
  Gain1/1 -> Simulink-PS Converter1/1
  PS-Simulink Converter1/1 -> Sum/1
  Sum/1 -> Gain/1
  Constant/1 -> Sum/2
  Saturation/1 -> Simulink-PS Converter2/1
  Gain/1 -> Saturation/1
  connections:
  Simulink-PS Converter2/RConn1 -- Ball Valve (IL)2/LConn2
  Ball Valve (IL)2/LConn1 -- Interface (TL-IL)2/RConn1
  Tank (IL)/LConn3 -- PS-Simulink Converter1/LConn1
  Ball Valve (IL)2/RConn1 -- Tank (IL)/LConn1
  Tank (IL)/LConn2 -- Ball Valve (IL)1/RConn1
  Simulink-PS Converter1/RConn1 -- Ball Valve (IL)1/LConn2
  Reservoir (IL)/LConn1 -- Ball Valve (IL)1/LConn1
  Cold Fluid/RConn1 -- Interface (TL-IL)2/LConn1

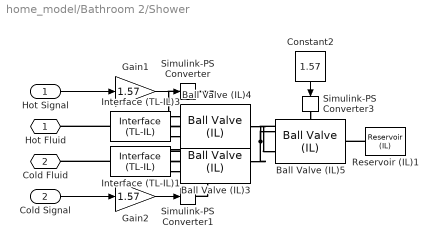
== system home_model/Bathroom 2/Shower ==
  Hot Signal : Inport
  Cold Signal : Inport  Port=2
  Ball Valve (IL)3 : SimscapeFluids_lib/Isothermal Liquid/Valves & Orifices/Flow Control Valves/Ball Valve (IL)  valve_type=fluids.isothermal_liquid.valves_orifices.flow_control_valves.enum.BallValveSpec.Standard  parameterization=fluids.isothermal_liquid.valves_orifices.flow_control_valves.enum.FlowCoefficientSpec.Kv  Cv_max=32 gpm  Kv_max=2 gpm  Cd=0.64  area_port=pi * (75 ^ 2) / 4 mm^2  area_ball=pi * (75 ^ 2) / 4 mm^2  Cv_TLU=[1e-06, .58, 1.15, 1.9, 2.8, 4.3, 7, 10.5, 17, 26, 32] gpm  Kv_TLU=[1e-06, .34, .76, 1.6, 2.45, 4.1, 5.75, 9.4, 13, 28, 50] m^3/hr  area_TLU=[1e-10, 62.5, 125, 187.5, 250, 312.5, 375, 437.5, 500, 562.5, 625] mm^2  rotation_TLU=pi / 2 .* [0, .1, .2, .3, .4, .5, .6, .7, .8, .9, 1] rad  area_leak=1e-10 m^2  Re_c=150  rho_water60F=0.99897 g/cm^3  rho_water15C=0.99913 g/cm^3
      settings: InternalSimscapePortConfiguration="{\"Bottom\":[],\"Left\":[{\"id\":\"A\",\"label\":\"A\",\"type\":\"foundation.isothermal_liquid.isothermal_liquid\"}],\"Right\":[{\"id\":\"B\",\"label\":\"B\",\"type\":\"foundation.isothermal_liquid.isothermal_liquid\"}],\"Top\":[{\"id\":\"S\",\"label\":\"S\",\"type\":\"input\"}]}"
  Ball Valve (IL)4 : SimscapeFluids_lib/Isothermal Liquid/Valves & Orifices/Flow Control Valves/Ball Valve (IL)  valve_type=fluids.isothermal_liquid.valves_orifices.flow_control_valves.enum.BallValveSpec.Standard  parameterization=fluids.isothermal_liquid.valves_orifices.flow_control_valves.enum.FlowCoefficientSpec.Kv  Cv_max=32 gpm  Kv_max=2 gpm  Cd=0.64  area_port=pi * (75 ^ 2) / 4 mm^2  area_ball=pi * (75 ^ 2) / 4 mm^2  Cv_TLU=[1e-06, .58, 1.15, 1.9, 2.8, 4.3, 7, 10.5, 17, 26, 32] gpm  Kv_TLU=[1e-06, .34, .76, 1.6, 2.45, 4.1, 5.75, 9.4, 13, 28, 50] m^3/hr  area_TLU=[1e-10, 62.5, 125, 187.5, 250, 312.5, 375, 437.5, 500, 562.5, 625] mm^2  rotation_TLU=pi / 2 .* [0, .1, .2, .3, .4, .5, .6, .7, .8, .9, 1] rad  area_leak=1e-10 m^2  Re_c=150  rho_water60F=0.99897 g/cm^3  rho_water15C=0.99913 g/cm^3
      settings: InternalSimscapePortConfiguration="{\"Bottom\":[],\"Left\":[{\"id\":\"A\",\"label\":\"A\",\"type\":\"foundation.isothermal_liquid.isothermal_liquid\"}],\"Right\":[{\"id\":\"B\",\"label\":\"B\",\"type\":\"foundation.isothermal_liquid.isothermal_liquid\"}],\"Top\":[{\"id\":\"S\",\"label\":\"S\",\"type\":\"input\"}]}"
  Ball Valve (IL)5 : SimscapeFluids_lib/Isothermal Liquid/Valves & Orifices/Flow Control Valves/Ball Valve (IL)  valve_type=fluids.isothermal_liquid.valves_orifices.flow_control_valves.enum.BallValveSpec.Standard  parameterization=fluids.isothermal_liquid.valves_orifices.flow_control_valves.enum.FlowCoefficientSpec.Kv  Cv_max=32 gpm  Kv_max=2 gpm  Cd=0.64  area_port=pi * (25 ^ 2) / 4 mm^2  area_ball=pi * (20 ^ 2) / 4 mm^2  Cv_TLU=[1e-06, .58, 1.15, 1.9, 2.8, 4.3, 7, 10.5, 17, 26, 32] gpm  Kv_TLU=[1e-06, .34, .76, 1.6, 2.45, 4.1, 5.75, 9.4, 13, 28, 50] m^3/hr  area_TLU=[1e-10, 62.5, 125, 187.5, 250, 312.5, 375, 437.5, 500, 562.5, 625] mm^2  rotation_TLU=pi / 2 .* [0, .1, .2, .3, .4, .5, .6, .7, .8, .9, 1] rad  area_leak=1e-10 m^2  Re_c=150  rho_water60F=0.99897 g/cm^3  rho_water15C=0.99913 g/cm^3
      settings: InternalSimscapePortConfiguration="{\"Bottom\":[],\"Left\":[{\"id\":\"A\",\"label\":\"A\",\"type\":\"foundation.isothermal_liquid.isothermal_liquid\"}],\"Right\":[{\"id\":\"B\",\"label\":\"B\",\"type\":\"foundation.isothermal_liquid.isothermal_liquid\"}],\"Top\":[{\"id\":\"S\",\"label\":\"S\",\"type\":\"input\"}]}"
  Constant2 : Constant  Value=1.57
  Gain1 : Gain  Gain=1.57
  Gain2 : Gain  Gain=1.57
  Interface (TL-IL)1 : SimscapeFluids_lib/Fluid Network Interfaces/Interface (TL-IL)  interface_domain_spec=fluids.interfaces.enum.interface_domain_spec.TL_IL  temperature_spec=foundation.enum.constant_controlled.constant  T_interface=293.15 K  area_TL=0.01 m^2
      settings: InternalSimscapePortConfiguration="{\"Bottom\":[],\"Left\":[{\"id\":\"TL\",\"label\":\"TL\",\"type\":\"foundation.thermal_liquid.thermal_liquid\"}],\"Right\":[{\"id\":\"IL\",\"label\":\"IL\",\"type\":\"foundation.isothermal_liquid.isothermal_liquid\"}],\"Top\":[]}"
  Interface (TL-IL)3 : SimscapeFluids_lib/Fluid Network Interfaces/Interface (TL-IL)  interface_domain_spec=fluids.interfaces.enum.interface_domain_spec.TL_IL  temperature_spec=foundation.enum.constant_controlled.constant  T_interface=293.15 K  area_TL=0.01 m^2
      settings: InternalSimscapePortConfiguration="{\"Bottom\":[],\"Left\":[{\"id\":\"TL\",\"label\":\"TL\",\"type\":\"foundation.thermal_liquid.thermal_liquid\"}],\"Right\":[{\"id\":\"IL\",\"label\":\"IL\",\"type\":\"foundation.isothermal_liquid.isothermal_liquid\"}],\"Top\":[]}"
  Reservoir (IL)1 : fl_lib/Isothermal Liquid/Elements/Reservoir (IL)  reservoir_type=foundation.enum.constant_controlled.constant  pressure_spec=foundation.enum.pressure_spec.atmospheric  reservoir_pressure=0.101325 MPa
  Simulink-PS Converter : nesl_utility/Simulink-PS Converter  PhysicalDomain=network_engine_domain  SubClassName=ps_input  LeftPortType=input  RightPortType=output  PseudoPeriodic=off  Frequencies=[]  NoiseDistribution=none  NoiseParameters=[]  Unit=1  AffineConversion=off  FilteringAndDerivatives=provide  SimscapeFilterOrder=1  InputFilterTimeConstant=0.001  UdotUserProvided=0
  Simulink-PS Converter1 : nesl_utility/Simulink-PS Converter  PhysicalDomain=network_engine_domain  SubClassName=ps_input  LeftPortType=input  RightPortType=output  PseudoPeriodic=off  Frequencies=[]  NoiseDistribution=none  NoiseParameters=[]  Unit=1  AffineConversion=off  FilteringAndDerivatives=provide  SimscapeFilterOrder=1  InputFilterTimeConstant=0.001  UdotUserProvided=0
  Simulink-PS Converter3 : nesl_utility/Simulink-PS Converter  PhysicalDomain=network_engine_domain  SubClassName=ps_input  LeftPortType=input  RightPortType=output  PseudoPeriodic=off  Frequencies=[]  NoiseDistribution=none  NoiseParameters=[]  Unit=1  AffineConversion=off  FilteringAndDerivatives=provide  SimscapeFilterOrder=1  InputFilterTimeConstant=0.001  UdotUserProvided=0
  Hot Fluid : PMIOPort  Side=Left
  Cold Fluid : PMIOPort  Port=2  Side=Left
  wires:
  Cold Signal/1 -> Gain2/1
  Gain2/1 -> Simulink-PS Converter1/1
  Gain1/1 -> Simulink-PS Converter/1
  Hot Signal/1 -> Gain1/1
  Constant2/1 -> Simulink-PS Converter3/1
  connections:
  Ball Valve (IL)3/LConn2 -- Simulink-PS Converter1/RConn1
  Simulink-PS Converter/RConn1 -- Ball Valve (IL)4/LConn2
  Interface (TL-IL)1/RConn1 -- Ball Valve (IL)3/LConn1
  Interface (TL-IL)1/LConn1 -- Cold Fluid/RConn1
  Interface (TL-IL)3/RConn1 -- Ball Valve (IL)4/LConn1
  Interface (TL-IL)3/LConn1 -- Hot Fluid/RConn1
  Reservoir (IL)1/LConn1 -- Ball Valve (IL)5/RConn1
  Simulink-PS Converter3/RConn1 -- Ball Valve (IL)5/LConn2
  Ball Valve (IL)4/RConn1 -- Ball Valve (IL)5/LConn1 -- Ball Valve (IL)3/RConn1
